simulink model "motor_pos"  (R2020b)
settings: Solver=ode15s  StartTime=0.0  StopTime=0.2  RelTol=1e-3
values from neighbouring files (symbols this model uses):
  b = 3.5077E-6    [motor_pos.sldd]
  J = 3.2284E-6    [motor_pos.sldd]
  K = 0.0274    [motor_pos.sldd]
  L = 2.75E-6    [motor_pos.sldd]
  R = 4.0    [motor_pos.sldd]
settings Model: Creator=priyaD  LastModifiedBy=priyaD

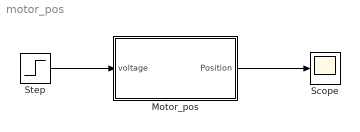
== system motor_pos ==
  Motor_pos : Subsystem
  Scope : Scope
  Step : Step  Time=0  SampleTime=0
  wires:
  Step/1 -> Motor_pos/1(voltage)
  Motor_pos/1(Position) -> Scope/1

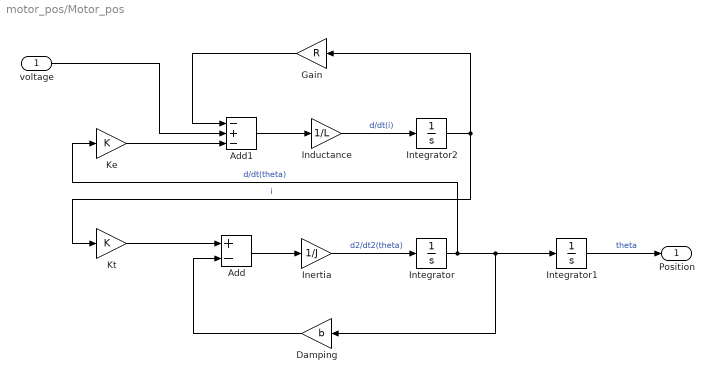
== system motor_pos/Motor_pos ==
  voltage : Inport
  Add : Sum  Inputs=+-
  Add1 : Sum  Inputs=-+-
  Damping : Gain  Gain=b
  Gain : Gain  Gain=R
  Inductance : Gain  Gain=1/L
  Inertia : Gain  Gain=1/J
  Integrator : Integrator
  Integrator1 : Integrator
  Integrator2 : Integrator
  Ke : Gain  Gain=K
  Kt : Gain  Gain=K
  Position : Outport
  wires:
  Damping/1 -> Add/2
  Inertia/1 -> Integrator/1  "d2/dt2(theta)"
  Integrator1/1 -> Position/1  "theta"
  Integrator/1 -> Ke/1, Damping/1, Integrator1/1  "d/dt(theta)"
  Integrator2/1 -> Gain/1, Kt/1  "i"
  Add/1 -> Inertia/1
  Kt/1 -> Add/1
  voltage/1 -> Add1/2
  Gain/1 -> Add1/1
  Inductance/1 -> Integrator2/1  "d/dt(i)"
  Ke/1 -> Add1/3
  Add1/1 -> Inductance/1
